simulink model "gm_MATE_HDLsolver_myFirstCircuit"  (R2024b)
settings: Solver=FixedStepDiscrete  StartTime=0.0  StopTime=0.05  FixedStep=6.02409638554217e-09  MaxStep=100e-6  RelTol=1e-4
PostLoadFcn:
  | Ts=1e-6; nb_sw=3; nb_lc=2;nb_r=1;nb_src=1; nb_out=3; rL=1.2;rC=100;L=1e-3; C=1e-5; LpejoSw=1e-6;h=Ts; MAX_INPUTS=16;
  | MAX_OUTPUTS=16;
  | MAX_SWITCHES=8;
  | MAX_INPUTS=16;
InitFcn:
  | Ts=1e-6; nb_sw=3; nb_lc=2;nb_r=1;nb_src=1; nb_out=3; rL=1.2;rC=100;L=1e-3; C=1e-5; LpejoSw=1e-6;h=Ts; MAX_INPUTS=16;
  | MAX_OUTPUTS=16;
  | MAX_SWITCHES=8;
  | MAX_INPUTS=16;
undefined symbols (not defined in the file or in its folder): MATE_SOC
libraries: fl_lib x31, nesl_utility x13, hdlmdlgenlib x10, simetranss x5, simulink x4, hdlsllib x3, ee_lib x2, eeGeneralControl x1
(part 1 of 8)
Description:
  | Copyright 2008-2010 The MathWorks, Inc.
settings Model: Creator=Kyle Diller
settings SolverCC: AlgebraicLoopSolver=TrustRegion
settings DataIOCC: SaveFormat=Array  SignalLoggingSaveFormat=ModelDataLogs  ReturnWorkspaceOutputs=off  SignalLoggingName=sigsOut
settings OptimizationCC: BlockReduction=off  ConditionallyExecuteInputs=off  OptimizeBlockIOStorage=off  BufferReuse=off  GlobalBufferReuse=off  ExpressionFolding=off  ExpressionDepthLimit=2147483647  LocalBlockOutputs=off  InitFltsAndDblsToZero=on  LifeSpan=inf
settings DebuggingCC: SaveWithParameterizedLinksMsg=none  UnderspecifiedInitializationDetection=Classic  MergeDetectMultiDrivingBlocksExec=none  CheckExecutionContextPreStartOutputMsg=on  SignalResolutionControl=TryResolveAllWithWarning  InheritedTsInSrcMsg=none  MultiTaskDSMMsg=warning  MultiTaskCondExecSysMsg=none  SingleTaskRateTransMsg=error  SigSpecEnsureSampleTimeMsg=none  FcnCallInpInsideContextMsg=warning  UnconnectedInputMsg=warning  UnconnectedOutputMsg=warning  UnconnectedLineMsg=warning  AllowSymbolicDim=off  StateNameClashWarn=warning  SFUnexpectedBacktrackingDiag=warning  SFNoUnconditionalDefaultTransitionDiag=warning  SFExecutionAtInitializationDiag=none  ArithmeticOperatorsInVariantConditions=warning
settings HardwareCC: ProdBitPerPointer=32  ProdBitPerSizeT=32  ProdBitPerPtrDiffT=32  ProdLargestAtomicFloat=None  ProdIntDivRoundTo=Undefined  ProdEndianess=Unspecified  ProdWordSize=32  ProdHWDeviceType=Specified  TargetUnknown=on
settings ModelReferenceCC: EnableRefExpFcnMdlSchedulingChecks=on  PropagateSignalLabelsOutOfModel=off
settings SFSimCC: SimUseLocalCustomCode=off  CustomCodeUndefinedFunction=UseInterfaceOnly
settings RTWCC: RTWUseLocalCustomCode=off  GPUComputeCapability=3.5
settings CodeAppCC: StateflowObjectComments=on
settings GRTTargetCC: TargetFcnLib=ansi_tfl_tmw.mat  TargetLangStandard=C89/C90 (ANSI)  CombineOutputUpdateFcns=off  GRTInterface=on
settings ConfigComp: CovMetricSettings=dw  CovSaveCumulativeToWorkspaceVar=on  CovSaveSingleToWorkspaceVar=on  CovExternalEMLEnable=off
settings SimscapeCC: SimscapeNormalizeSystem=off

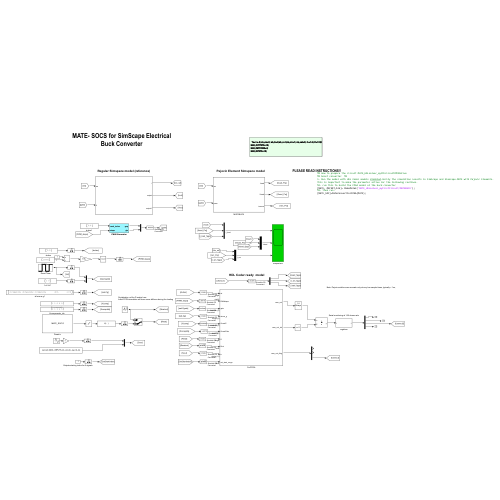
[thumbnail: Simulink's stored preview of the top-level diagram]
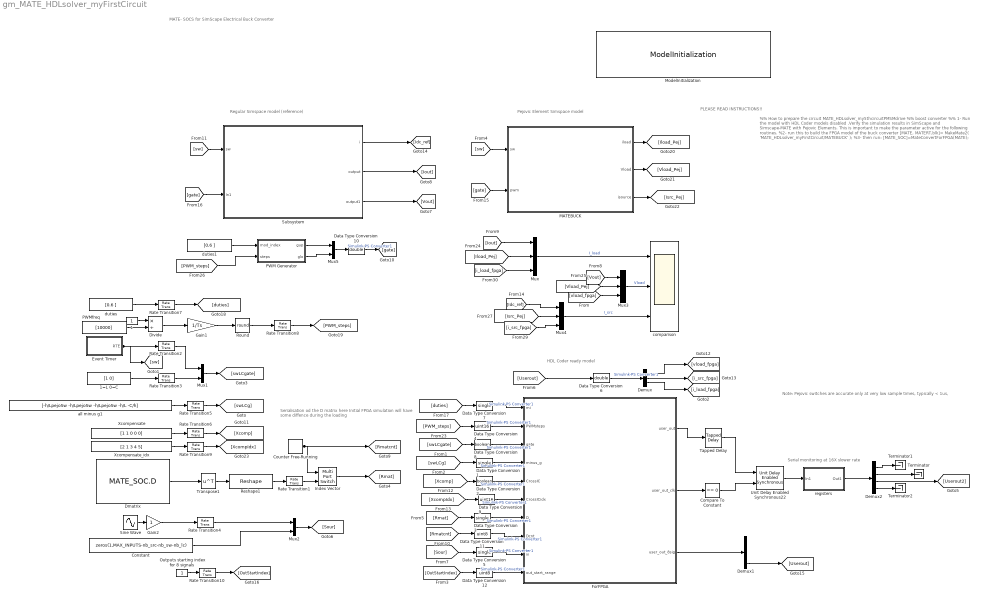
== system gm_MATE_HDLsolver_myFirstCircuit ==
  note: MATE- SOCS for SimScape Electrical
      | Buck Converter
  note: HDL Coder ready model
  note: %% How to prepare the circuit MATE_HDLsolver_my5thcircuitPMSMdrive
      | %% boost converter %%
      | 1- Run the model with HDL Coder models disabled .Verify the simulation results in SimScape and Simscape-MATE with Pejovic Elements.
      | This is important to make the parameter active for the following routines.
      | %2- run this to build the FPGA model of the buck converter
      | [MATE, MATERT,blk]= MakeMate2( 'MATE_HDLsolver_myFirstCircuit/MATEBUCK' );
      | %3- then run:
      | [MATE_SOC]=MateConvertForFPGA(MATE);
  note: PLEASE READ INSTRUCTIONS!!
  note: Pejovic Element Simspace model
  note: Note: Pejovic switches are accurate only at very low sample times, typically < 1us,
  note: Regular Simspace model (reference)
  note: Serialisation od the D matrix here
      | Initial FPGA simulation will have some diffence during the loading
  note: Serial monitoring at 16X slower rate
  " Event Timer" : Subsystem  Tag=RTEcontrol_s38shd7k88  LoadFcn=|  mask(Timer){is=0 (off), t=[0.01 0.02 0.03 0.04 ], Tmax=0.07, Ts=Ts}
      | xx=get_param(gcb,'linkstatus');      
      | if isequal(xx,'inactive')            
      | set_param(gcb,'linkstatus','restore')
      | end
      mask prompts: is "Initial state"; t "Transition times (s):"; Tmax "Repeat period (s)"; Ts "Sample time (s)"
      mask help: This block generates a Simulink control signal changing at specified transition times.
      mask init:
      | iss=get_param(gcb,'is');
      | if isequal(iss,'0 (off)')
      |     sw(1)=0;
      |     sw(2)=0;
      | else
      |     sw(1)=1;
      |     sw(2)=1;
      | end
      | st(1)=0;
      | st(2)=t(1);
      | 
      | if t(1)==0,
      |    h=errordlg(' The first time specified must be greater than 0 ' , 'Parameter error');
      | end
      | 
      | i=3;
      | tog=0;
      | ptr=2;
      | while length(sw)<=2*length(t)
      |     if tog==0
      |         st=[st st(end)+Ts];
      |         sw=[sw 1-sw(end)];
      |         tog=1;
      |     else
      |         st=[st t(ptr)];
      |         sw=[sw sw(end)];
      |         ptr=ptr+1;
      |         tog=0;
      |     end
      | 
      | end
      |  %st=[st Tmax-Ts Tmax+Ts]
      | % sw=[sw sw(end) sw(1)]
      mask TypeOptions is: 0 (off) | 1 (on)
      mask Display:
      | %plot(0,0,100,100,[70,40,40,20,20,13],[30,30,70,70,30,30]);
      | plot( st(1:end-1), sw(1:end-1) );
  1 : Constant
  1=L 0=C : Constant  Value=[1 0]
  Compare To Constant : hdlsllib/Logic and Bit Operations/Compare To Constant  relop===  const=0  OutDataTypeStr=boolean
  Constant : Constant  Value=zeros(1,MAX_INPUTS-nb_src-nb_sw-nb_lc)
  Counter Free-Running : hdlsllib/Sources/Counter Free-Running  NumBits=8  tsamp=-1
  Data Type Conversion{1,3,5,7} (4 alike) : DataTypeConversion  OutDataTypeStr=single  RndMeth=Nearest  SaturateOnIntegerOverflow=off
  Data Type Conversion10 : DataTypeConversion  OutDataTypeStr=double  RndMeth=Nearest  SaturateOnIntegerOverflow=off
  Data Type Conversion11 : DataTypeConversion  OutDataTypeStr=uint8  RndMeth=Nearest  SaturateOnIntegerOverflow=off
  Data Type Conversion12 : DataTypeConversion  OutDataTypeStr=uint8  RndMeth=Nearest  SaturateOnIntegerOverflow=off
  Data Type Conversion2 : DataTypeConversion  OutDataTypeStr=boolean  RndMeth=Nearest  SaturateOnIntegerOverflow=off
  Data Type Conversion4 : DataTypeConversion  OutDataTypeStr=uint16  RndMeth=Nearest  SaturateOnIntegerOverflow=off
  Data Type Conversion6 : DataTypeConversion  OutDataTypeStr=double  RndMeth=Nearest  SaturateOnIntegerOverflow=off
  Data Type Conversion8 : DataTypeConversion  OutDataTypeStr=boolean  RndMeth=Nearest  SaturateOnIntegerOverflow=off
  Data Type Conversion9 : DataTypeConversion  OutDataTypeStr=uint16  RndMeth=Nearest  SaturateOnIntegerOverflow=off
  Demux : Demux  Outputs=3
  Demux1 : Demux  Outputs=[nb_sw nb_lc nb_out ]
  Demux2 : Demux  Outputs=[nb_sw nb_lc nb_out MAX_OUTPUTS-nb_out-nb_sw-nb_lc]
  Divide : Product  Inputs=*/
  Dmatrix : Constant  Value=MATE_SOC.D
  ForFPGA : Subsystem
  Gain1 : Gain  Gain=1/Ts
  Gain2 : Gain
  Index Vector : MultiPortSwitch  DataPortOrder=Zero-based contiguous  Inputs=1  zeroidx=on  SaturateOnIntegerOverflow=off  InputSameDT=off
  MATEBUCK : Subsystem
  ModelInitialization : simetranss/Usefulls/ModelInitialization  InitFcnX=|  prel=off  posl=on  inif=on  strf=off
      | Ts=1e-6; nb_sw=3; nb_lc=2;nb_r=1;nb_src=1; nb_out=3; rL=1.2;rC=100;L=1e-3; C=1e-5; LpejoSw=1e-6;h=Ts; MAX_INPUTS=16;
      | MAX_OUTPUTS=16;
      | MAX_SWITCHES=8;
      | MAX_INPUTS=16;
  Mux : Mux  Inputs=3
  Mux1 : Mux  Inputs=2
  Mux2 : Mux  Inputs=2
  Mux3 : Mux  Inputs=3
  Mux4 : Mux  Inputs=3
  Mux5 : Mux  Inputs=2
  Outputs starting index for 8 signals : Constant
  PWM Generator : Subsystem  Tag=RTEcontrol_s38shd7k88
  PWMfreq : Constant  Value=[10000]
  Rate Transition{1..10} (10 alike) : RateTransition  OutPortSampleTime=1e-06
  Reshape1 : Reshape
  Round : Rounding  Operator=round
  Sine Wave : Sin  Amplitude=0  Bias=100  Frequency=0  SampleTime=0
  Subsystem : Subsystem
  Tapped Delay : simulink/Discrete/Tapped Delay  vinit=0.0  samptime=-1  NumDelays=16  DelayOrder=Oldest  includeCurrent=off
      settings: LibrarySourceBlock=hdlsllib/Discrete/Tapped Delay
  Terminator : Terminator
  Terminator1 : Terminator
  Terminator2 : Terminator
  Transpose1 : Math  Operator=transpose
  Unit Delay Enabled Synchronous22 : hdlsllib/Discrete/Unit Delay Enabled Synchronous  InitialCondition=0.0  SampleTime=-1
  Xcompensate : Constant  Value=[1 1 0 0 0]
  Xcompensate_idx : Constant  Value=[2 1 3 4 5]
  all minus g1 : Constant  Value=[-h/LpejoSw -h/LpejoSw -h/LpejoSw -h/L -C/h]
  comparison : Scope  NumInputPorts=3
  duties : Constant  Value=[0.6 ]
  duties1 : Constant  Value=[0.6 ]
  registers : Subsystem
  wires:
  [sw] -> Subsystem/1(sw)
  Outputs starting index for 8 signals/1 -> Rate Transition10/1
  Rate Transition10/1 -> [OutStartIndex]
  Data Type Conversion12/1 -> ForFPGA/10(out_start_range)  "Simulink-PS Converter1"
  [OutStartIndex] -> Data Type Conversion12/1
  Demux1/3 -> [Userout]
  ForFPGA/3(user_out_8sig) -> Demux1/1
  registers/1(Out1) -> Demux2/1
  Unit Delay Enabled Synchronous22/1 -> registers/1(In1)
  Compare To Constant/1 -> Unit Delay Enabled Synchronous22/2
  ForFPGA/1(user_out) -> Tapped Delay/1
  ForFPGA/2(user_out_clk) -> Compare To Constant/1
  Tapped Delay/1 -> Unit Delay Enabled Synchronous22/1
  Subsystem/3(output1) -> [Vout]
  Subsystem/2(output) -> [Iout]
  Subsystem/1(i) -> [Idc_ref]
  [gate] -> Subsystem/2(In1)
  Data Type Conversion7/1 -> ForFPGA/1(mi)  "Simulink-PS Converter1"
  Data Type Conversion11/1 -> ForFPGA/8(Dcnt)  "Simulink-PS Converter1"
  Data Type Conversion4/1 -> ForFPGA/2(PWMsteps)  "Simulink-PS Converter1"
  Data Type Conversion9/1 -> ForFPGA/6(CrossICidx)  "Simulink-PS Converter1"
  Data Type Conversion1/1 -> ForFPGA/4(minus_g)  "Simulink-PS Converter1"
  [PWM_steps] -> Data Type Conversion4/1
  Data Type Conversion3/1 -> ForFPGA/7(D)  "Simulink-PS Converter1"
  Data Type Conversion5/1 -> ForFPGA/9(in)  "Simulink-PS Converter1"
  Data Type Conversion2/1 -> ForFPGA/5(CrossIC)  "Simulink-PS Converter1"
  Data Type Conversion8/1 -> ForFPGA/3(gate)  "Simulink-PS Converter1"
  [duties] -> Data Type Conversion7/1
  [Rmat] -> Data Type Conversion3/1
  [Sour] -> Data Type Conversion5/1
  [Xcomp] -> Data Type Conversion2/1
  [swLCgate] -> Data Type Conversion8/1
  [XcompIdx] -> Data Type Conversion9/1
  [swLCg] -> Data Type Conversion1/1
  [Rmatcnt] -> Data Type Conversion11/1
  Index Vector/1 -> [Rmat]
  Counter Free-Running/1 -> [Rmatcnt], Index Vector/1
  Rate Transition1/1 -> Index Vector/2
  Reshape1/1 -> Rate Transition1/1
  Transpose1/1 -> Reshape1/1
  [Iout] -> Mux/1
  Data Type Conversion10/1 -> [gate]  "Simulink-PS Converter1"
  Mux5/1 -> Data Type Conversion10/1
  PWM Generator/1(gup) -> Mux5/1
  PWM Generator/2(glo) -> Mux5/2
  [PWM_steps] -> PWM Generator/2(steps)
  duties1/1 -> PWM Generator/1(mod_index)
  Round/1 -> Rate Transition8/1
  Rate Transition9/1 -> [XcompIdx]
  Xcompensate_idx/1 -> Rate Transition9/1
  [i_src_fpga] -> Mux4/3
  Demux/3 -> [i_load_fpga]
  1/1 -> Divide/1
  PWMfreq/1 -> Divide/2
  Demux2/4 -> Terminator2/1
  Demux2/1 -> Terminator1/1
  Demux2/3 -> [Userout2]
  [Isrc_Pej] -> Mux4/2
  [Idc_ref] -> Mux4/1
  Mux4/1 -> comparison/3  "I_src"
  [Vload_Pej] -> Mux3/2
  [i_load_fpga] -> Mux/3
  [Iload_Pej] -> Mux/2
  MATEBUCK/3(isource) -> [Isrc_Pej]
  MATEBUCK/2(Vload) -> [Vload_Pej]
  MATEBUCK/1(iload) -> [Iload_Pej]
  Demux2/2 -> Terminator/1
  Gain1/1 -> Round/1
  Divide/1 -> Gain1/1
  Rate Transition8/1 -> [PWM_steps]
  Constant/1 -> Mux2/2
  Rate Transition4/1 -> Mux2/1
  Mux2/1 -> [Sour]
  Rate Transition7/1 -> [duties]
  duties/1 -> Rate Transition7/1
  [gate] -> MATEBUCK/2(pwm)
  Data Type Conversion6/1 -> Demux/1  "Simulink-PS Converter1"
  [vload_fpga] -> Mux3/3
  Demux/2 -> [i_src_fpga]
  Demux/1 -> [vload_fpga]
  Xcompensate/1 -> Rate Transition6/1
  Rate Transition6/1 -> [Xcomp]
  Gain2/1 -> Rate Transition4/1
  Rate Transition5/1 -> [swLCg]
  all minus g1/1 -> Rate Transition5/1
  Mux1/1 -> [swLCgate]
  [sw] -> MATEBUCK/1(sw)
  [Vout] -> Mux3/1
  Mux3/1 -> comparison/2  "Vload"
  Rate Transition3/1 -> Mux1/2
  1=L 0=C/1 -> Rate Transition3/1
  [Userout] -> Data Type Conversion6/1
  Sine Wave/1 -> Gain2/1
  Rate Transition2/1 -> Mux1/1
  " Event Timer"/1(RTE) -> Rate Transition2/1, [sw]
  Dmatrix/1 -> Transpose1/1
  Mux/1 -> comparison/1  "I_load"

== system gm_MATE_HDLsolver_myFirstCircuit/ Event Timer ==
  Repeating Sequence : simulink/Sources/Repeating Sequence  rep_seq_t=st  rep_seq_y=sw
  Repeating Sequence1 : simulink/Sources/Repeating Sequence  Commented=on  rep_seq_t="[0    0.2000    0.2001    0.4000    0.4001    0.6000    2.0000]"  rep_seq_y=|
      | [     1     1     0     0     1     1     1
      | ]
  RTE : Outport  VectorParamsAs1DForOutWhenUnconnected=off
  wires:
  Repeating Sequence/1 -> RTE/1
